simulink model "Tariq"  (Simulink 7.3)
settings: Solver=ode45  StartTime=0.0  StopTime=10  RelTol=1e-3
values from neighbouring files (symbols this model uses):
  B = 0.01    [Induction.m]
  f = 50    [Induction.m]
  J = 1.662    [Induction.m]
  Lm = 0.04    [Induction.m]
  Lr = 0.043    [Induction.m]
  Ls = 0.0425    [Induction.m]
  P = 4    [Induction.m]
  Rr = 0.187    [Induction.m]
  Rs = 0.087    [Induction.m]
  Vm = sqrt(2)*Vph    [Induction.m]
  We = 2*pi*50    (= 314.159265359)    [Induction.m]
libraries: simulink x2
settings Model: Creator=Administrator  LastModifiedBy=ASAD
settings OptimizationCC: InitFltsAndDblsToZero=on
settings DebuggingCC: SaveWithParameterizedLinksMsg=none  SignalResolutionControl=TryResolveAllWithWarning
settings GRTTargetCC: TargetFcnLib=ansi_tfl_tmw.mat

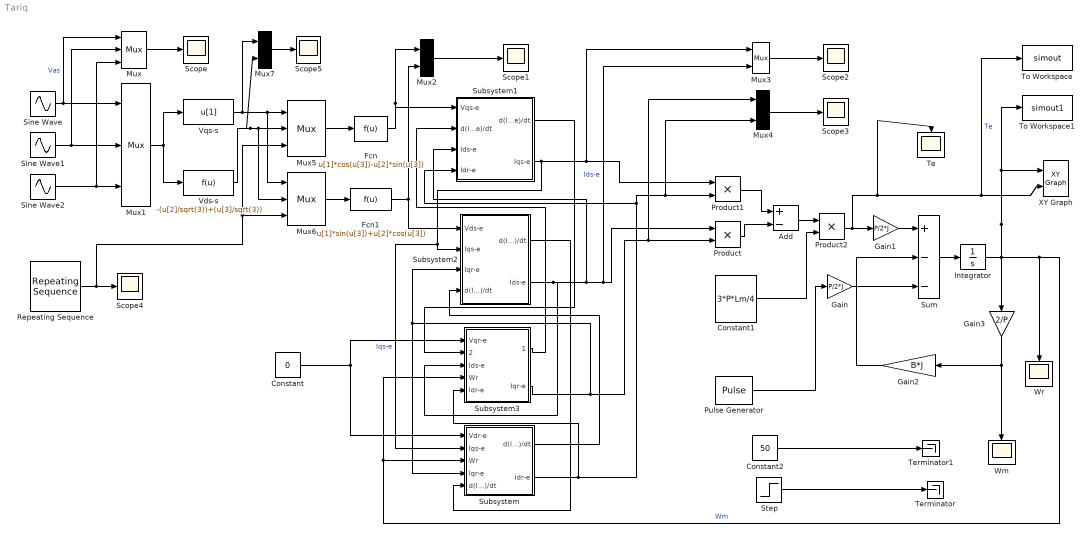
== system Tariq ==
  Add : Sum  Inputs=+-  OutDataType=sfix(16)  OutScaling=2^-10
  Constant : Constant  Value=0  OutDataType=sfix(16)  OutScaling=2^0
  Constant1 : Constant  Value=3*P*Lm/4  OutDataType=sfix(16)  OutScaling=2^0
  Constant2 : Constant  Value=50  OutDataType=sfix(16)  OutScaling=2^0
  Fcn : Fcn  Expr=u[1]*cos(u[3])-u[2]*sin(u[3])
  Fcn1 : Fcn  Expr=u[1]*sin(u[3])+u[2]*cos(u[3])
  Gain : Gain  Gain=P/2*J  ParameterDataType=sfix(16)  ParameterScaling=2^0  OutDataType=sfix(16)  OutScaling=2^0
  Gain1 : Gain  Gain=P/2*J  ParameterDataType=sfix(16)  ParameterScaling=2^0  OutDataType=sfix(16)  OutScaling=2^0
  Gain2 : Gain  Gain=B*J  ParameterDataType=sfix(16)  ParameterScaling=2^0  OutDataType=sfix(16)  OutScaling=2^0
  Gain3 : Gain  Gain=2/P  ParameterDataType=sfix(16)  ParameterScaling=2^0  OutDataType=sfix(16)  OutScaling=2^0
  Integrator : Integrator
  Mux{,1,5..6} (4 alike) : Mux  Inputs=3
      settings: DisplayOption=signals
  Mux{2..4,7} (4 alike) : Mux  Inputs=2
      settings: DisplayOption=signals
  Product : Product  OutDataType=sfix(16)  OutScaling=2^0  RndMeth=Zero
  Product1 : Product  OutDataType=sfix(16)  OutScaling=2^0  RndMeth=Zero
  Product2 : Product  OutDataType=sfix(16)  OutScaling=2^0  RndMeth=Zero
  Pulse Generator : DiscretePulseGenerator  Amplitude=40  Period=10  PulseWidth=5  PhaseDelay=4  SampleTime=1
  Repeating Sequence : simulink/Sources/Repeating Sequence  SystemSampleTime=-1  rep_seq_t=[0 1/f]  rep_seq_y=[0 2*pi]
  Scope{,1..5} (6 alike) : Scope
      Scope settings: YMin=-400  YMax=350
      Scope1 settings: YMin=-25  YMax=400
      Scope2 settings: SaveName=ScopeData2
      Scope3 settings: YMin=-2e+006  YMax=1.1e+007  SaveName=ScopeData3
      Scope4 settings: SaveName=ScopeData5
      Scope5 settings: YMin=-400  YMax=0  SaveName=ScopeData6
  Sine Wave : Sin  Amplitude=Vm  Bias=0  Frequency=2*pi*50  Phase=pi/2  Samples=10  SampleTime=0  Offset=0
  Sine Wave1 : Sin  Amplitude=Vm  Bias=0  Frequency=2*pi*50  Phase=(pi/2)-(2*pi/3)  Samples=10  SampleTime=0  Offset=0
  Sine Wave2 : Sin  Amplitude=Vm  Bias=0  Frequency=2*pi*50  Phase=(pi/2)+(2*pi/3)  Samples=10  SampleTime=0  Offset=0
  Step : Step  Time=0.5  After=40  SampleTime=0
  Subsystem : Subsystem
  Subsystem1 : Subsystem
  Subsystem2 : Subsystem
  Subsystem3 : Subsystem
  Sum : Sum  Inputs=+--  OutDataType=sfix(16)  OutScaling=2^0
  Te : Scope
      settings: SaveName=ScopeData8
  Terminator : Terminator
  Terminator1 : Terminator
  To Workspace : ToWorkspace  VariableName=simout  SampleTime=-1  SaveFormat=Structure
  To Workspace1 : ToWorkspace  VariableName=simout1  SampleTime=-1  SaveFormat=Structure
  Vds-s : Fcn  Expr=-(u[2]/sqrt(3))+(u[3]/sqrt(3))
  Vqs-s : Fcn  Expr=u[1]
  Wm : Scope
      settings: YMin=-1250  YMax=1500  SaveName=ScopeData4
  Wr : Scope
      settings: YMax=400  SaveName=ScopeData7
  XY Graph : simulink/Sinks/XY Graph  SystemSampleTime=-1  xmin=0  xmax=350  ymin=-400  ymax=400  st=-1
  wires:
  Mux/1 -> Scope/1
  Mux2/1 -> Scope1/1
  Mux3/1 -> Scope2/1
  Mux4/1 -> Scope3/1
  Product1/1 -> Add/1
  Product/1 -> Add/2
  Add/1 -> Product2/1
  Constant1/1 -> Product2/2
  Product2/1 -> Gain1/1, XY Graph/2, To Workspace/1, Te/1  "Te"
  Gain1/1 -> Sum/1
  Gain/1 -> Sum/3
  Pulse Generator/1 -> Gain/1
  Sum/1 -> Integrator/1
  Integrator/1 -> XY Graph/1, To Workspace1/1, Gain3/1, Subsystem3/4(Wr), Subsystem/3(Wr), Wr/1  "Wm"
  Gain2/1 -> Sum/2
  Gain3/1 -> Wm/1, Gain2/1
  Constant2/1 -> Terminator1/1
  Step/1 -> Terminator/1
  Repeating Sequence/1 -> Scope4/1, Mux5/3, Mux6/3
  Sine Wave/1 -> Mux1/1, Mux/1  "Vas"
  Sine Wave1/1 -> Mux1/2, Mux/2
  Sine Wave2/1 -> Mux1/3, Mux/3
  Mux1/1 -> Vqs-s/1, Vds-s/1
  Vqs-s/1 -> Mux5/1, Mux6/1, Mux7/1
  Vds-s/1 -> Mux5/2, Mux6/2, Mux7/2
  Mux5/1 -> Fcn/1
  Mux6/1 -> Fcn1/1
  Fcn/1 -> Mux2/1, Subsystem1/1(Vqs-e)
  Fcn1/1 -> Mux2/2, Subsystem2/1(Vds-e)
  Mux7/1 -> Scope5/1
  Subsystem1/2(Iqs-e) -> Subsystem2/2(Iqs-e), Subsystem/2(Iqs-e), Product1/1, Mux3/1  "Iqs-e"
  Subsystem/2(Idr-e) -> Subsystem1/4(Idr-e), Product1/2, Mux4/2, Subsystem3/5(Idr-e)
  Subsystem2/2(Ids-e) -> Subsystem1/3(Ids-e), Product/1, Mux3/2, Subsystem3/3(Ids-e)  "Ids-e"
  Subsystem3/2(Iqr-e) -> Subsystem2/3(Iqr-e), Subsystem/4(Iqr-e), Product/2, Mux4/1
  Subsystem/1(d(Idr-e)/dt) -> Subsystem2/4(d(Idr-e)/dt)
  Constant/1 -> Subsystem3/1(Vqr-e), Subsystem/1(Vdr-e)
  Subsystem1/1(d(Iqs-e)/dt) -> Subsystem3/2(d(Iqs-e)/dt)
  Subsystem2/1(d(Ids-e)/dt) -> Subsystem/5(d(Ids-e)/dt)
  Subsystem3/1(d(Iqr-e)/dt) -> Subsystem1/2(d(Iqr-e)/dt)

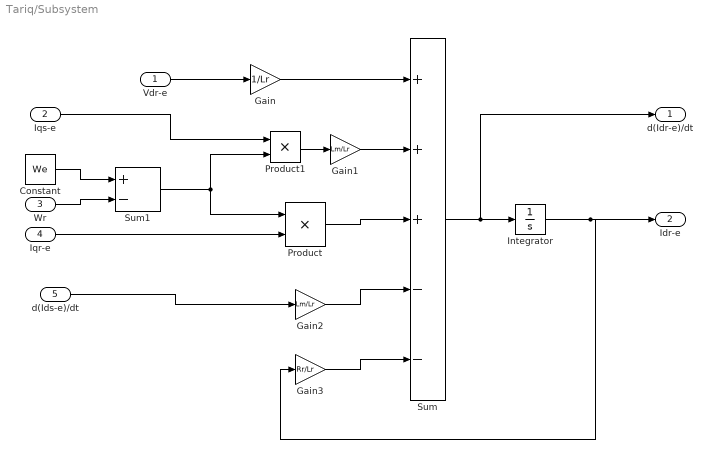
== system Tariq/Subsystem ==
  Vdr-e : Inport  OutDataType=sfix(16)  OutScaling=2^0
  Iqs-e : Inport  Port=2  OutDataType=sfix(16)  OutScaling=2^0
  Wr : Inport  Port=3  OutDataType=sfix(16)  OutScaling=2^0
  Iqr-e : Inport  Port=4  OutDataType=sfix(16)  OutScaling=2^0
  d(Ids-e)/dt : Inport  Port=5  OutDataType=sfix(16)  OutScaling=2^0
  Constant : Constant  Value=We  OutDataType=fixdt(1, 16)  OutScaling=2^0
  Gain : Gain  Gain=1/Lr  ParameterDataType=sfix(16)  ParameterScaling=2^0  OutDataType=sfix(16)  OutScaling=2^0
  Gain1 : Gain  Gain=Lm/Lr  ParameterDataType=sfix(16)  ParameterScaling=2^0  OutDataType=sfix(16)  OutScaling=2^0
  Gain2 : Gain  Gain=Lm/Lr  ParameterDataType=sfix(16)  ParameterScaling=2^0  OutDataType=sfix(16)  OutScaling=2^0
  Gain3 : Gain  Gain=Rr/Lr  ParameterDataType=sfix(16)  ParameterScaling=2^0  OutDataType=sfix(16)  OutScaling=2^0
  Integrator : Integrator
  Product : Product  OutDataType=sfix(16)  OutScaling=2^0  RndMeth=Zero
  Product1 : Product  OutDataType=sfix(16)  OutScaling=2^0  RndMeth=Zero
  Sum : Sum  Inputs=+++--  OutDataType=sfix(16)  OutScaling=2^0
  Sum1 : Sum  Inputs=+-  OutDataType=sfix(16)  OutScaling=2^0
  d(Idr-e)/dt : Outport  OutDataType=sfix(16)  OutScaling=2^0
  Idr-e : Outport  Port=2  OutDataType=sfix(16)  OutScaling=2^0
  wires:
  Gain/1 -> Sum/1
  Vdr-e/1 -> Gain/1
  Gain1/1 -> Sum/2
  Product1/1 -> Gain1/1
  Sum1/1 -> Product1/2, Product/1
  Constant/1 -> Sum1/1
  Wr/1 -> Sum1/2
  Iqs-e/1 -> Product1/1
  Iqr-e/1 -> Product/2
  Product/1 -> Sum/3
  Gain2/1 -> Sum/4
  d(Ids-e)/dt/1 -> Gain2/1
  Sum/1 -> Integrator/1, d(Idr-e)/dt/1
  Integrator/1 -> Idr-e/1, Gain3/1
  Gain3/1 -> Sum/5

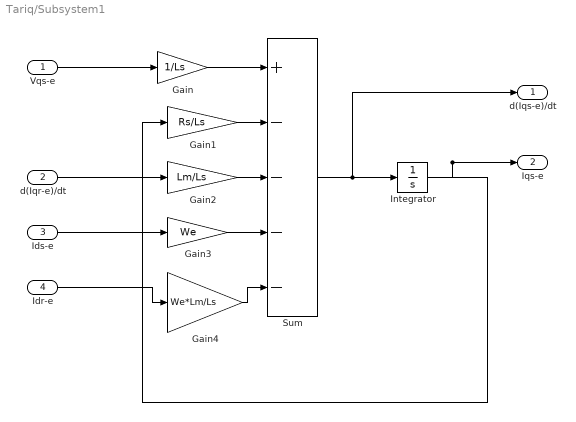
== system Tariq/Subsystem1 ==
  Vqs-e : Inport  OutDataType=sfix(16)  OutScaling=2^0
  d(Iqr-e)/dt : Inport  Port=2  OutDataType=sfix(16)  OutScaling=2^0
  Ids-e : Inport  Port=3  OutDataType=sfix(16)  OutScaling=2^0
  Idr-e : Inport  Port=4  OutDataType=sfix(16)  OutScaling=2^0
  Gain : Gain  Gain=1/Ls  ParameterDataType=sfix(16)  ParameterScaling=2^0  OutDataType=sfix(16)  OutScaling=2^0
  Gain1 : Gain  Gain=Rs/Ls  ParameterDataType=sfix(16)  ParameterScaling=2^0  OutDataType=sfix(16)  OutScaling=2^0
  Gain2 : Gain  Gain=Lm/Ls  ParameterDataType=sfix(16)  ParameterScaling=2^0  OutDataType=sfix(16)  OutScaling=2^0
  Gain3 : Gain  Gain=We  ParameterDataType=sfix(16)  ParameterScaling=2^0  OutDataType=sfix(16)  OutScaling=2^0
  Gain4 : Gain  Gain=We*Lm/Ls  ParameterDataType=sfix(16)  ParameterScaling=2^0  OutDataType=sfix(16)  OutScaling=2^0
  Integrator : Integrator
  Sum : Sum  Inputs=+----  OutDataType=sfix(16)  OutScaling=2^0
  d(Iqs-e)/dt : Outport  OutDataType=sfix(16)  OutScaling=2^0
  Iqs-e : Outport  Port=2  OutDataType=sfix(16)  OutScaling=2^0
  wires:
  Vqs-e/1 -> Gain/1
  Gain/1 -> Sum/1
  Gain1/1 -> Sum/2
  Gain2/1 -> Sum/3
  Sum/1 -> Integrator/1, d(Iqs-e)/dt/1
  d(Iqr-e)/dt/1 -> Gain2/1
  Integrator/1 -> Iqs-e/1, Gain1/1
  Gain3/1 -> Sum/4
  Ids-e/1 -> Gain3/1
  Gain4/1 -> Sum/5
  Idr-e/1 -> Gain4/1

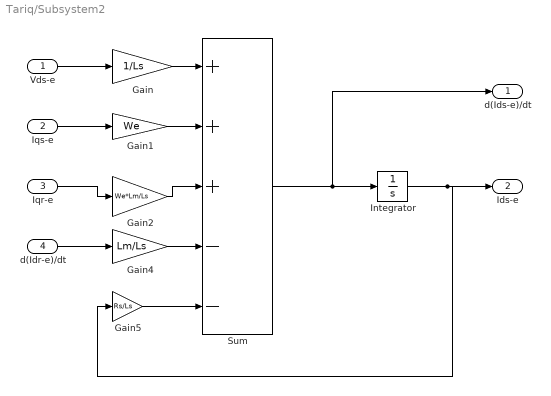
== system Tariq/Subsystem2 ==
  Vds-e : Inport  OutDataType=sfix(16)  OutScaling=2^0
  Iqs-e : Inport  Port=2  OutDataType=sfix(16)  OutScaling=2^0
  Iqr-e : Inport  Port=3  OutDataType=sfix(16)  OutScaling=2^0
  d(Idr-e)/dt : Inport  Port=4  OutDataType=sfix(16)  OutScaling=2^0
  Gain : Gain  Gain=1/Ls  ParameterDataType=sfix(16)  ParameterScaling=2^0  OutDataType=sfix(16)  OutScaling=2^0
  Gain1 : Gain  Gain=We  ParameterDataType=sfix(16)  ParameterScaling=2^0  OutDataType=sfix(16)  OutScaling=2^0
  Gain2 : Gain  Gain=We*Lm/Ls  ParameterDataType=sfix(16)  ParameterScaling=2^0  OutDataType=sfix(16)  OutScaling=2^0
  Gain4 : Gain  Gain=Lm/Ls  ParameterDataType=sfix(16)  ParameterScaling=2^0  OutDataType=sfix(16)  OutScaling=2^0
  Gain5 : Gain  Gain=Rs/Ls  ParameterDataType=sfix(16)  ParameterScaling=2^0  OutDataType=sfix(16)  OutScaling=2^0
  Integrator : Integrator
  Sum : Sum  Inputs=+++--  OutDataType=sfix(16)  OutScaling=2^0
  d(Ids-e)/dt : Outport  OutDataType=sfix(16)  OutScaling=2^0
  Ids-e : Outport  Port=2  OutDataType=sfix(16)  OutScaling=2^0
  wires:
  Gain/1 -> Sum/1
  Vds-e/1 -> Gain/1
  Gain1/1 -> Sum/2
  Iqs-e/1 -> Gain1/1
  Iqr-e/1 -> Gain2/1
  Gain2/1 -> Sum/3
  d(Idr-e)/dt/1 -> Gain4/1
  Gain4/1 -> Sum/4
  Gain5/1 -> Sum/5
  Sum/1 -> Integrator/1, d(Ids-e)/dt/1
  Integrator/1 -> Ids-e/1, Gain5/1

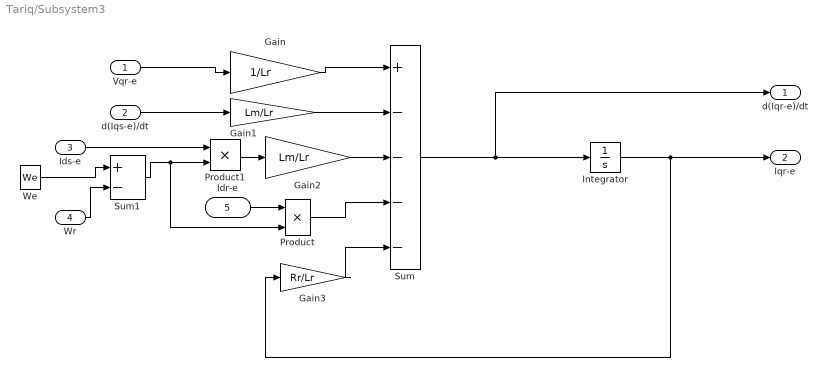
== system Tariq/Subsystem3 ==
  Vqr-e : Inport  OutDataType=sfix(16)  OutScaling=2^0
  d(Iqs-e)/dt : Inport  Port=2  OutDataType=sfix(16)  OutScaling=2^0
  Ids-e : Inport  Port=3  OutDataType=sfix(16)  OutScaling=2^0
  Wr : Inport  Port=4  OutDataType=sfix(16)  OutScaling=2^0
  Idr-e : Inport  Port=5  OutDataType=sfix(16)  OutScaling=2^0
  Gain : Gain  Gain=1/Lr  ParameterDataType=sfix(16)  ParameterScaling=2^0  OutDataType=sfix(16)  OutScaling=2^0
  Gain1 : Gain  Gain=Lm/Lr  ParameterDataType=sfix(16)  ParameterScaling=2^0  OutDataType=sfix(16)  OutScaling=2^0
  Gain2 : Gain  Gain=Lm/Lr  ParameterDataType=sfix(16)  ParameterScaling=2^0  OutDataType=sfix(16)  OutScaling=2^0
  Gain3 : Gain  Gain=Rr/Lr  ParameterDataType=sfix(16)  ParameterScaling=2^0  OutDataType=sfix(16)  OutScaling=2^0
  Integrator : Integrator
  Product : Product  OutDataType=sfix(16)  OutScaling=2^0  RndMeth=Zero
  Product1 : Product  OutDataType=sfix(16)  OutScaling=2^0  RndMeth=Zero
  Sum : Sum  Inputs=+----  OutDataType=sfix(16)  OutScaling=2^0
  Sum1 : Sum  Inputs=+-  OutDataType=sfix(16)  OutScaling=2^0
  We : Constant  Value=We  OutDataType=fixdt(1, 16)  OutScaling=2^0
  d(Iqr-e)/dt : Outport  OutDataType=sfix(16)  OutScaling=2^0
  Iqr-e : Outport  Port=2  OutDataType=sfix(16)  OutScaling=2^0
  wires:
  Gain/1 -> Sum/1
  Gain1/1 -> Sum/2
  Sum/1 -> Integrator/1, d(Iqr-e)/dt/1
  Integrator/1 -> Iqr-e/1, Gain3/1
  Vqr-e/1 -> Gain/1
  d(Iqs-e)/dt/1 -> Gain1/1
  Ids-e/1 -> Product1/1
  Product1/1 -> Gain2/1
  Gain2/1 -> Sum/3
  Sum1/1 -> Product1/2, Product/2
  Wr/1 -> Sum1/2
  Product/1 -> Sum/4
  Idr-e/1 -> Product/1
  Gain3/1 -> Sum/5
  We/1 -> Sum1/1
